simulink subsystem "rss_ElecSpdCtlSenl"  (R2023a)
settings: Solver=VariableStepAuto  StartTime=0.0  StopTime=10.0  RelTol=1e-3
undefined symbols (not defined in the file): bit, Cdbl_nElecAgSpdMaxVal, Cdbl_trqTqMaxVal, ENM_MOTO_STATUS, Gs16_trqInitCondTq_C
libraries: lib_configurable_parameter x2, simulink x1, lib_discrete_time_PI_controller x1, lib_discrete_time_PI_controller32bit x1
settings Model: DefaultTestHarness=rss_ElectricSpeedController_SensorLess_thu  Creator=RAN2OFO  LastModifiedBy=xiaoqiang.yuan
settings OptimizationCC: ReuseModelBlockBuffer=off

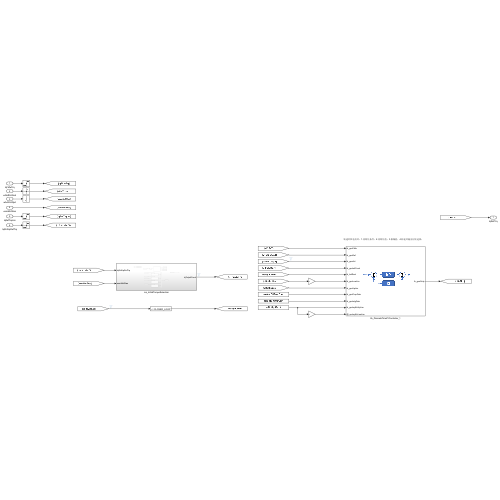
[thumbnail: Simulink's stored preview of the top-level diagram]
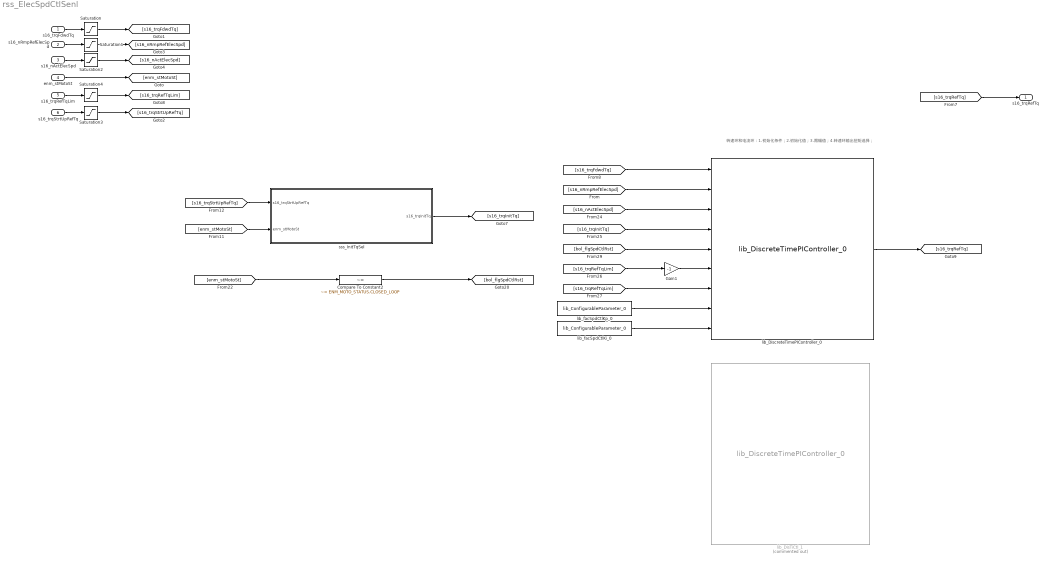
== system rss_ElecSpdCtlSenl ==
  note: 转速环和电流环：1.初始化条件；2.初始化值；3.限幅值；4.转速环输出扭矩选择；
  s16_trqFdwdTq : Inport  OutDataTypeStr=dt_Standardize_s16p15b0
  s16_nRmpRefElecSpd : Inport  Port=2  OutDataTypeStr=dt_Standardize_s16p15b0
  s16_nActElecSpd : Inport  Port=3  OutDataTypeStr=dt_Standardize_s16p15b0
  enm_stMotoSt : Inport  Port=4  OutDataTypeStr=Enum: ENM_MOTO_STATUS
  s16_trqRefTqLim : Inport  Port=5  OutDataTypeStr=dt_Standardize_s16p15b0
  s16_trqStrtUpRefTq : Inport  Port=6  OutDataTypeStr=dt_Standardize_s16p15b0
  Compare To Constant2 : simulink/Logic and Bit Operations/Compare To Constant  relop=~=  const=ENM_MOTO_STATUS.CLOSED_LOOP  OutDataTypeStr=boolean
  Gain1 : Gain  Gain=-1  RndMeth=Simplest  OutDataTypeStr=Inherit: Same as input
  Saturation : Saturate  UpperLimit=Cdbl_trqTqMaxVal  LowerLimit=-Cdbl_trqTqMaxVal
  Saturation1 : Saturate  UpperLimit=Cdbl_nElecAgSpdMaxVal  LowerLimit=-Cdbl_nElecAgSpdMaxVal
  Saturation2 : Saturate  UpperLimit=Cdbl_nElecAgSpdMaxVal  LowerLimit=-Cdbl_nElecAgSpdMaxVal
  Saturation3 : Saturate  UpperLimit=Cdbl_trqTqMaxVal  LowerLimit=-Cdbl_trqTqMaxVal
  Saturation4 : Saturate  UpperLimit=Cdbl_trqTqMaxVal  LowerLimit=-Cdbl_trqTqMaxVal
  lib_DisTiCtl_1 : lib_discrete_time_PI_controller/lib_DiscreteTimePIController_0  Commented=on  lb_parSampTime=Cu16_tiSlwTaskSmpTi  lb_parMaxSampTime=0.1  lb_parMaxPropGain=Cdbl_facSpdCtlKpMaxVal  lb_parMaxIntgGain=Cdbl_facSpdCtlKiMaxVal  lb_parRefInpMaxVal=Cdbl_nElecAgSpdMaxVal  lb_parRefInpMinVal=-Cdbl_nElecAgSpdMaxVal  lb_parMaxErrVal=2*Cdbl_nElecAgSpdMaxVal  lb_parMinErrVal=-2*Cdbl_nElecAgSpdMaxVal  lb_parMaxOutpVal=Cdbl_trqTqMaxVal  lb_parMinOutpVal=-Cdbl_trqTqMaxVal  lb_parAccmDataTypeMode=32-bit  lb_parOutpDataType=dt_Standardize_s16p15b0  lb_parSatMode=anti-windup with back-calculation
  lib_DiscreteTimePIController_0 : lib_discrete_time_PI_controller32bit/lib_DiscreteTimePIController_0  lb_parSampTime=Cdbl_tiSlwTaskSmpTi  lb_parMaxSampTime=0.1  lb_parMaxPropGain=Cdbl_facSpdCtlKpMaxVal  lb_parMaxIntgGain=Cdbl_facSpdCtlKiMaxVal  lb_parRefInpMaxVal=Cdbl_nElecAgSpdMaxVal  lb_parRefInpMinVal=-Cdbl_nElecAgSpdMaxVal  lb_parMaxErrVal=2*Cdbl_nElecAgSpdMaxVal  lb_parMinErrVal=-2*Cdbl_nElecAgSpdMaxVal  lb_parMaxOutpVal=Cdbl_trqTqMaxVal  lb_parMinOutpVal=-Cdbl_trqTqMaxVal  lb_parAccmDataTypeMode=32-bit  lb_parOutpDataType=dt_Standardize_s16p15b0  lb_parSatMode=anti-windup with back-calculation
  lib_facSpdCtlKi_0 : lib_configurable_parameter/lib_ConfigurableParameter_0  lb_parCnfgPar=Gu16_facSpdCtlKi_C  lb_parDataType=Inherit: Inherit from 'Constant value'  lb_parUpLim=Cdbl_facSpdCtlKiMaxVal  lb_parLowLim=0
  lib_facSpdCtlKp_0 : lib_configurable_parameter/lib_ConfigurableParameter_0  lb_parCnfgPar=Gu16_facSpdCtlKp_C  lb_parDataType=Inherit: Inherit from 'Constant value'  lb_parUpLim=Cdbl_facSpdCtlKpMaxVal  lb_parLowLim=0
  sss_InitTqSel : Subsystem  VariantControl=cstSensCtrlLbl
  s16_trqRefTq : Outport  OutDataTypeStr=dt_Standardize_s16p15b0
  wires:
  s16_trqFdwdTq/1 -> Saturation/1
  s16_trqRefTqLim/1 -> Saturation4/1
  enm_stMotoSt/1 -> [enm_stMotoSt]
  Saturation4/1 -> [s16_trqRefTqLim]
  Saturation1/1 -> [s16_nRmpRefElecSpd]
  s16_nRmpRefElecSpd/1 -> Saturation1/1
  s16_nActElecSpd/1 -> Saturation2/1
  [s16_trqRefTq] -> s16_trqRefTq/1
  Saturation2/1 -> [s16_nActElecSpd]
  Saturation/1 -> [s16_trqFdwdTq]
  Compare To Constant2/1 -> [bol_flgSpdCtlRst]
  [s16_nActElecSpd] -> lib_DiscreteTimePIController_0/3
  [s16_nRmpRefElecSpd] -> lib_DiscreteTimePIController_0/2
  [s16_trqInitTq] -> lib_DiscreteTimePIController_0/4
  lib_DiscreteTimePIController_0/1 -> [s16_trqRefTq]
  [s16_trqRefTqLim] -> Gain1/1
  Gain1/1 -> lib_DiscreteTimePIController_0/6
  [s16_trqRefTqLim] -> lib_DiscreteTimePIController_0/7
  sss_InitTqSel/1(s16_trqInitTq) -> [s16_trqInitTq]
  [s16_trqStrtUpRefTq] -> sss_InitTqSel/1(s16_trqStrtUpRefTq)
  [enm_stMotoSt] -> sss_InitTqSel/2(enm_stMotoSt)
  s16_trqStrtUpRefTq/1 -> Saturation3/1
  Saturation3/1 -> [s16_trqStrtUpRefTq]
  [enm_stMotoSt] -> Compare To Constant2/1
  lib_facSpdCtlKp_0/1 -> lib_DiscreteTimePIController_0/8
  lib_facSpdCtlKi_0/1 -> lib_DiscreteTimePIController_0/9
  [bol_flgSpdCtlRst] -> lib_DiscreteTimePIController_0/5
  [s16_trqFdwdTq] -> lib_DiscreteTimePIController_0/1

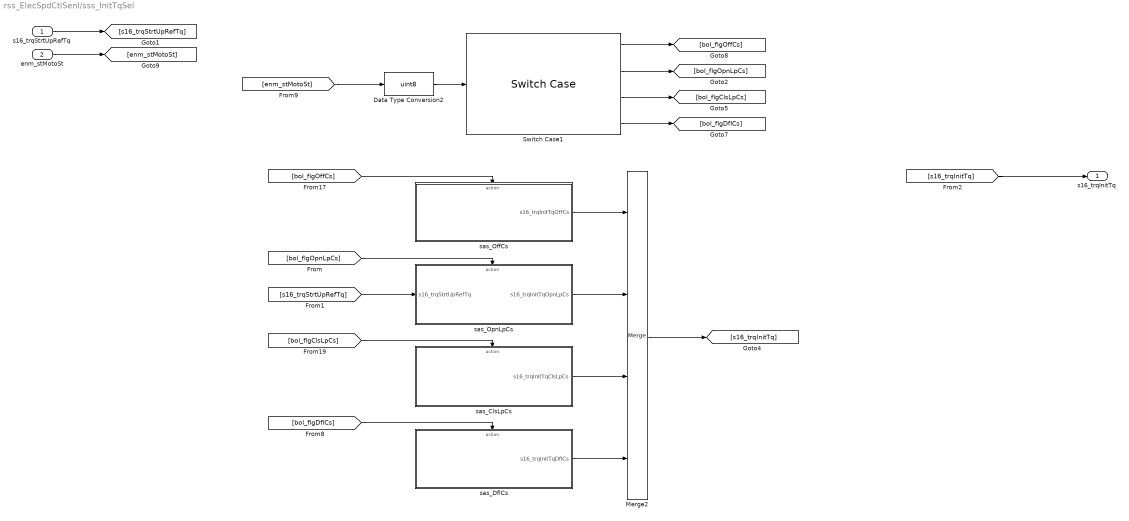
== system rss_ElecSpdCtlSenl/sss_InitTqSel ==
  s16_trqStrtUpRefTq : Inport
  enm_stMotoSt : Inport  Port=2
  Data Type Conversion2 : DataTypeConversion  OutDataTypeStr=uint8  SaturateOnIntegerOverflow=off  RndMeth=Floor
  Merge2 : Merge  Inputs=4
  Switch Case1 : SwitchCase  CaseConditions={0,1,2}
  sas_ClsLpCs : Subsystem  TreatAsAtomicUnit=on
  sas_DflCs : Subsystem  TreatAsAtomicUnit=on
  sas_OffCs : Subsystem  TreatAsAtomicUnit=on
  sas_OpnLpCs : Subsystem  TreatAsAtomicUnit=on
  s16_trqInitTq : Outport
  wires:
  Switch Case1/3 -> [bol_flgClsLpCs]
  Switch Case1/2 -> [bol_flgOpnLpCs]
  [s16_trqStrtUpRefTq] -> sas_OpnLpCs/1(s16_trqStrtUpRefTq)
  [bol_flgClsLpCs] -> sas_ClsLpCs/Action
  sas_ClsLpCs/1(s16_trqInitTqClsLpCs) -> Merge2/3
  sas_DflCs/1(s16_trqInitTqDflCs) -> Merge2/4
  sas_OpnLpCs/1(s16_trqInitTqOpnLpCs) -> Merge2/2
  s16_trqStrtUpRefTq/1 -> [s16_trqStrtUpRefTq]
  Switch Case1/1 -> [bol_flgOffCs]
  Merge2/1 -> [s16_trqInitTq]
  [bol_flgOpnLpCs] -> sas_OpnLpCs/Action
  [bol_flgDflCs] -> sas_DflCs/Action
  sas_OffCs/1(s16_trqInitTqOffCs) -> Merge2/1
  [bol_flgOffCs] -> sas_OffCs/Action
  Data Type Conversion2/1 -> Switch Case1/1
  [enm_stMotoSt] -> Data Type Conversion2/1
  Switch Case1/4 -> [bol_flgDflCs]
  enm_stMotoSt/1 -> [enm_stMotoSt]
  [s16_trqInitTq] -> s16_trqInitTq/1

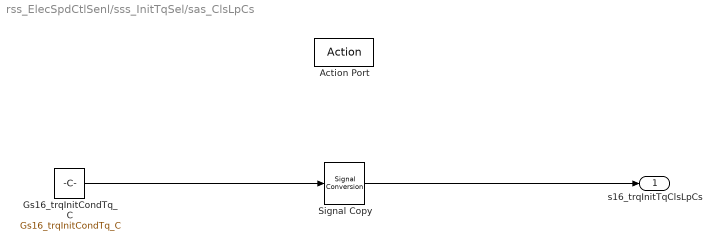
== system rss_ElecSpdCtlSenl/sss_InitTqSel/sas_ClsLpCs ==
  Action Port : ActionPort
  Gs16_trqInitCondTq_C : Constant  Value=Gs16_trqInitCondTq_C
  Signal Copy : SignalConversion  OverrideOpt=off
  s16_trqInitTqClsLpCs : Outport
  wires:
  Signal Copy/1 -> s16_trqInitTqClsLpCs/1
  Gs16_trqInitCondTq_C/1 -> Signal Copy/1

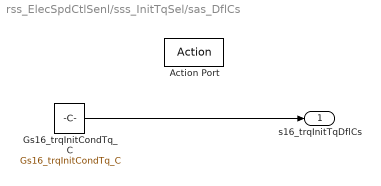
== system rss_ElecSpdCtlSenl/sss_InitTqSel/sas_DflCs ==
  Action Port : ActionPort
  Gs16_trqInitCondTq_C : Constant  Value=Gs16_trqInitCondTq_C
  s16_trqInitTqDflCs : Outport
  wires:
  Gs16_trqInitCondTq_C/1 -> s16_trqInitTqDflCs/1

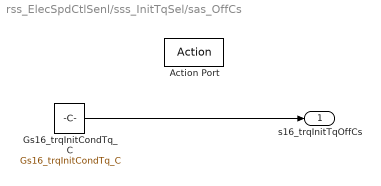
== system rss_ElecSpdCtlSenl/sss_InitTqSel/sas_OffCs ==
  Action Port : ActionPort
  Gs16_trqInitCondTq_C : Constant  Value=Gs16_trqInitCondTq_C
  s16_trqInitTqOffCs : Outport
  wires:
  Gs16_trqInitCondTq_C/1 -> s16_trqInitTqOffCs/1

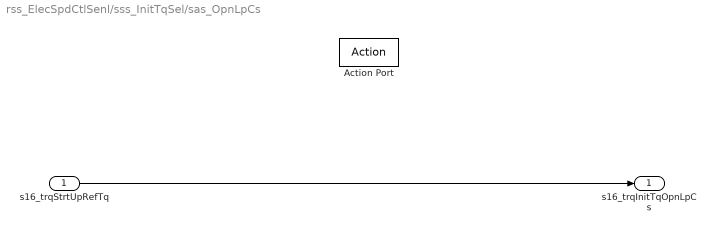
== system rss_ElecSpdCtlSenl/sss_InitTqSel/sas_OpnLpCs ==
  s16_trqStrtUpRefTq : Inport
  Action Port : ActionPort
  s16_trqInitTqOpnLpCs : Outport
  wires:
  s16_trqStrtUpRefTq/1 -> s16_trqInitTqOpnLpCs/1
